simulink model "ball_and_beam"  (R2014b)
settings: Solver=ode45  StartTime=0.0  StopTime=1  RelTol=1e-3
values from neighbouring files (symbols this model uses):
  Bm = 0.01    [ball.m]    (also in ball_and_beam.m; tham_so.m)
  g = 9.8    [ball.m]    (also in ball_and_beam.m; tham_so.m)
  Jb = (1/3)*mB*l^2    (= 0.00154666666667)    [ball.m]    (also in ball_and_beam.m = 0.0178133333333; parameter.m = (1/3)*mb*L^2; tham_so.m = 0.0178133333333)
  JB = (2/5)*mB*rB^2    (= 1.0469e-06)    [ball.m]    (also in ball_and_beam.m; parameter.m = (2/5)*mB*R^2; tham_so.m)
  Jm = 0.000052    (= 5.2e-05)    [ball.m]    (also in ball_and_beam.m; tham_so.m)
  Ke = 0.235    [ball.m]    (also in ball_and_beam.m; tham_so.m)
  Kt = 0.235    [ball.m]    (also in ball_and_beam.m; tham_so.m)
  La = 0.23    [ball.m]    (also in ball_and_beam.m; tham_so.m)
  Lb = 0.4    [tham_so.m]
  mb = 0.334    [ball.m]    (also in ball_and_beam.m; parameter.m; tham_so.m)
  mB = 0.029    [ball.m]    (also in ball_and_beam.m; parameter.m; tham_so.m)
  Ra = 2    [ball.m]    (also in ball_and_beam.m; tham_so.m)
  rB = 0.0095    [ball.m]    (also in ball_and_beam.m; tham_so.m)
settings Model: Creator=Admin  LastModifiedBy=Admin

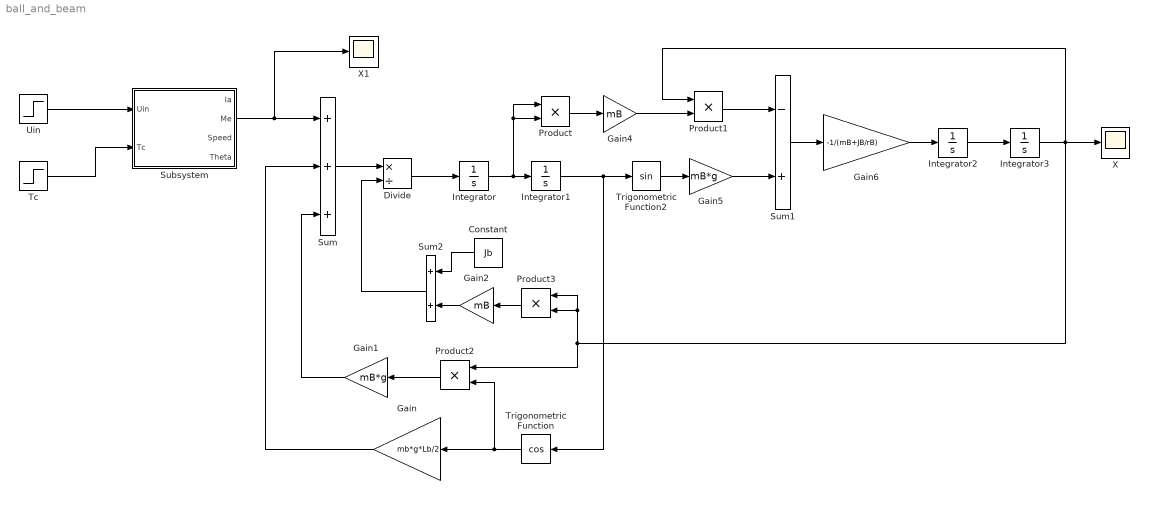
== system ball_and_beam ==
  Constant : Constant  Value=Jb
  Divide : Product  Inputs=*/
  Gain : Gain  Gain=mb*g*Lb/2
  Gain1 : Gain  Gain=mB*g
  Gain2 : Gain  Gain=mB
  Gain4 : Gain  Gain=mB
  Gain5 : Gain  Gain=mB*g
  Gain6 : Gain  Gain=-1/(mB+JB/rB)
  Integrator{,1..3} (4 alike) : Integrator
  Product{,1..3} (4 alike) : Product
  Subsystem : Subsystem
  Sum : Sum  Inputs=+++
  Sum1 : Sum  Inputs=-+
  Sum2 : Sum
  Tc : Step  Time=0  After=0  SampleTime=0
  Trigonometric Function : Trigonometry  Operator=cos
  Trigonometric Function2 : Trigonometry
  Uin : Step  Time=0  After=-1  SampleTime=0
  X : Scope
  X1 : Scope
  wires:
  Uin/1 -> Subsystem/1(Uin)
  Tc/1 -> Subsystem/2(Tc)
  Trigonometric Function/1 -> Product2/2, Gain/1
  Subsystem/2(Me) -> X1/1, Sum/1
  Gain/1 -> Sum/2
  Integrator/1 -> Product/2, Product/1, Integrator1/1
  Integrator1/1 -> Trigonometric Function2/1, Trigonometric Function/1
  Product/1 -> Gain4/1
  Trigonometric Function2/1 -> Gain5/1
  Gain5/1 -> Sum1/2
  Sum1/1 -> Gain6/1
  Integrator2/1 -> Integrator3/1
  Gain6/1 -> Integrator2/1
  Integrator3/1 -> Product3/2, Product3/1, Product2/1, Product1/1, X/1
  Gain4/1 -> Product1/2
  Product1/1 -> Sum1/1
  Product2/1 -> Gain1/1
  Gain1/1 -> Sum/3
  Product3/1 -> Gain2/1
  Gain2/1 -> Sum2/2
  Constant/1 -> Sum2/1
  Sum2/1 -> Divide/2
  Sum/1 -> Divide/1
  Divide/1 -> Integrator/1

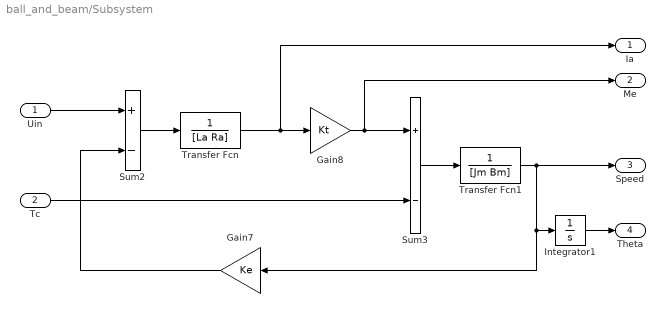
== system ball_and_beam/Subsystem ==
  Uin : Inport
  Tc : Inport  Port=2
  Gain7 : Gain  Gain=Ke
  Gain8 : Gain  Gain=Kt
  Integrator1 : Integrator
  Sum2 : Sum  Inputs=+-
  Sum3 : Sum  Inputs=+-
  Transfer Fcn : TransferFcn  Denominator=[La Ra]
  Transfer Fcn1 : TransferFcn  Denominator=[Jm Bm]
  Ia : Outport
  Me : Outport  Port=2
  Speed : Outport  Port=3
  Theta : Outport  Port=4
  wires:
  Gain7/1 -> Sum2/2
  Sum2/1 -> Transfer Fcn/1
  Gain8/1 -> Me/1, Sum3/1
  Transfer Fcn/1 -> Ia/1, Gain8/1
  Uin/1 -> Sum2/1
  Tc/1 -> Sum3/2
  Integrator1/1 -> Theta/1
  Sum3/1 -> Transfer Fcn1/1
  Transfer Fcn1/1 -> Gain7/1, Integrator1/1, Speed/1
